simulink model "DSTATCOM (1)"  (R2023b)
settings: Solver=ode5  StartTime=0.0  StopTime=1  FixedStep=50e-8  RelTol=1e-3
InitFcn:
  | v= 400
  | p= 2500
  | q=1500
  | s=2915.47
libraries: spsThreePhaseVIMeasurementLib x11, spsThreePhaseSeriesRLCBranchLib x9, spsThreePhaseSeriesRLCLoadLib x8, spsIGBTDiodeLib x6, slpidlib x4, spsRMSLib x2, spsAlphaBetaZerotodq0Lib x2, spsabctodq0Lib x2, spsSeriesRLCBranchLib x1, simulink x1, spsVoltageMeasurementLib x1, spsabctoAlphaBetaZeroLib x1
settings Model: Creator=prabh  LastModifiedBy=Sandesh

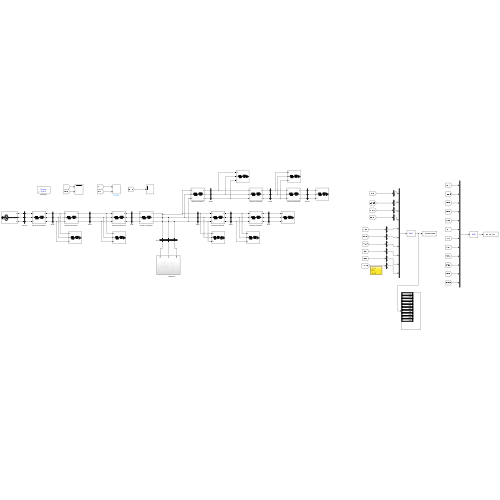
[thumbnail: Simulink's stored preview of the top-level diagram]
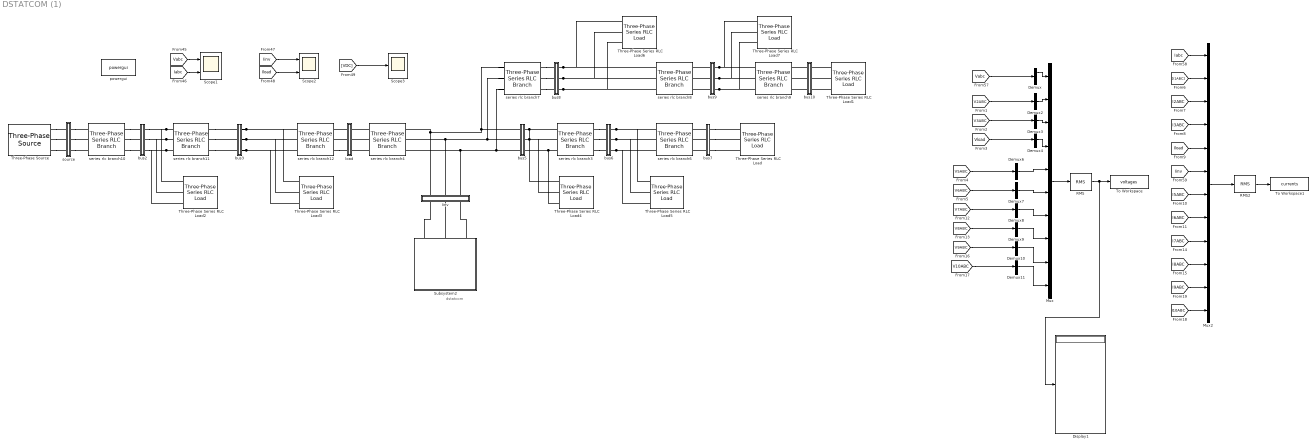
== system DSTATCOM (1) ==
  note: dstatcom
  Demux{,2..4,6..11} (10 alike) : Demux  Outputs=3
  Display1 : Display
  Iinv : Subsystem
  Mux : Mux  Inputs=10
  Mux2 : Mux  Inputs=12
  RMS : spsRMSLib/RMS  TrueRMS=on  Freq=50  RMSInit=0  Ts=0
  RMS2 : spsRMSLib/RMS  TrueRMS=on  Freq=50  RMSInit=0  Ts=0
  Scope1 : Scope  NumInputPorts=2
  Scope2 : Scope  NumInputPorts=2
  Scope3 : Scope
  Subsystem2 : Subsystem
  Three-Phase Series RLC Load{,1..3,5..7} (7 alike) : spsThreePhaseSeriesRLCLoadLib/Three-Phase Series RLC Load  LConnTagsString=A|B|C  Configuration=Y (grounded)  NominalVoltage=v  Vabc=[1e3 1e3 1e3]  Vabcp=[1e3 1e3 1e3]  NominalFrequency=50  UnbalancedPower=off  ActivePower=p  InductivePower=q  CapacitivePower=0  Pabc=[10e3 9e3 11e3]  QLabc=[100 90 110]  QCabc=[100 90 110]  Pabcp=[10e3 9e3 11e3]  QLabcp=[100 90 110]  QCabcp=[100 90 110]  Measurements=None  LoadType=constant PQ
  Three-Phase Series RLC Load4 : spsThreePhaseSeriesRLCLoadLib/Three-Phase Series RLC Load  LConnTagsString=A|B|C  Configuration=Y (grounded)  NominalVoltage=v  Vabc=[1e3 1e3 1e3]  Vabcp=[1e3 1e3 1e3]  NominalFrequency=50  UnbalancedPower=off  ActivePower=p  InductivePower=q  CapacitivePower=q  Pabc=[10e3 9e3 11e3]  QLabc=[100 90 110]  QCabc=[100 90 110]  Pabcp=[10e3 9e3 11e3]  QLabcp=[100 90 110]  QCabcp=[100 90 110]  Measurements=None  LoadType=constant PQ
  Three-Phase Source : spsThreePhaseSourceLib/Three-Phase Source  InternalConnection=Yg  VoltagePhases=off  Voltage=400  PhaseAngle=0  Voltage_phases=[25e3 25e3 25e3]/sqrt(3)  PhaseAngles_phases=[0 -120 +120]  Frequency=50  NonIdealSource=off  SpecifyImpedance=off  Resistance=0.8929  Inductance=16.58e-3  ShortCircuitLevel=100e6  BaseVoltage=25e3  XRratio=7  BusType=swing  Pref=10e3  Qref=0  Prefabc=[10e3, 10e3, 10e3]  Qrefabc=[0, 0, 0]  Qmin=-inf  Qmax=inf
  To Workspace : ToWorkspace  VariableName=voltages  SampleTime=-1
      settings: MaxDataPoints=1
  To Workspace1 : ToWorkspace  VariableName=currents  SampleTime=-1
      settings: MaxDataPoints=1
  bus10 : Subsystem
  bus2 : Subsystem
  bus3 : Subsystem
  bus5 : Subsystem
  bus6 : Subsystem
  bus7 : Subsystem
  bus8 : Subsystem
  bus9 : Subsystem
  load : Subsystem
  powergui : sps_lib/powergui  Priority=1  SimulationMode=Discrete  SampleTime=50e-6  frequency=60  Iterations=50  frequencyindice=0  Pbase=100e6  ErrMax=1e-4  UnitsV=kV  UnitsW=MW  buscounter=0  FunctionMessages=off  echomessages=off  EnableUseOfTLC=off  CurrentSourceSwitches=off  DisableSnubberDevices=off  DisableRonSwitches=off  DisableVfSwitches=off  DisplayEquations=off  AutomaticDiscreteSolvers=off  SolverType=Tustin/Backward Euler (TBE)  Interpol=off  ExternalGateDelay=off  methode=off  Ts=100  x0status=blocks  SPID=on  SwTol=0  HookPort=off  NonlinearTolerance=1e-4  nMaxIteration=100  ContinueOnMaxIteration=off  RestoreLinks=warning  ResistiveCurrentMeasurement=off  Frange=[0:2:500]  Ylog=off  Xlog=on  ShowGrid=off  save=off  variable=ZData  structure=0  ZoomFFT=off  StartTime=0.0  cycles=1  DisplayStyle=1  fundamental=60  FreqAxis=off  MaxFrequency=1000  frequencyindicesteady=1  RmsSteady=1  display=off
  series rlc branch10 : spsThreePhaseSeriesRLCBranchLib/Three-Phase Series RLC Branch  LConnTagsString=A|B|C  RConnTagsString=A|B|C  BranchType=RL  Resistance=0.3  Inductance=0.00027  Capacitance=0  Measurements=None
  series rlc branch11 : spsThreePhaseSeriesRLCBranchLib/Three-Phase Series RLC Branch  LConnTagsString=A|B|C  RConnTagsString=A|B|C  BranchType=RL  Resistance=.3  Inductance=.00177  Capacitance=0  Measurements=None
  series rlc branch12 : spsThreePhaseSeriesRLCBranchLib/Three-Phase Series RLC Branch  LConnTagsString=A|B|C  RConnTagsString=A|B|C  BranchType=RL  Resistance=.3  Inductance=.00218  Capacitance=0  Measurements=None
  series rlc branch3 : spsThreePhaseSeriesRLCBranchLib/Three-Phase Series RLC Branch  LConnTagsString=A|B|C  RConnTagsString=A|B|C  BranchType=RL  Resistance=.36  Inductance=.000821  Capacitance=0  Measurements=None
  series rlc branch4 : spsThreePhaseSeriesRLCBranchLib/Three-Phase Series RLC Branch  LConnTagsString=A|B|C  RConnTagsString=A|B|C  BranchType=RL  Resistance=.77  Inductance=.00218  Capacitance=0  Measurements=None
  series rlc branch6 : spsThreePhaseSeriesRLCBranchLib/Three-Phase Series RLC Branch  LConnTagsString=A|B|C  RConnTagsString=A|B|C  BranchType=RL  Resistance=.3  Inductance=.00068  Capacitance=0  Measurements=None
  series rlc branch7 : spsThreePhaseSeriesRLCBranchLib/Three-Phase Series RLC Branch  LConnTagsString=A|B|C  RConnTagsString=A|B|C  BranchType=RL  Resistance=.18  Inductance=.00041  Capacitance=0  Measurements=None
  series rlc branch8 : spsThreePhaseSeriesRLCBranchLib/Three-Phase Series RLC Branch  LConnTagsString=A|B|C  RConnTagsString=A|B|C  BranchType=RL  Resistance=.12  Inductance=.00027  Capacitance=0  Measurements=None
  series rlc branch9 : spsThreePhaseSeriesRLCBranchLib/Three-Phase Series RLC Branch  LConnTagsString=A|B|C  RConnTagsString=A|B|C  BranchType=RL  Resistance=.6  Inductance=.00136  Capacitance=0  Measurements=None
  source : Subsystem
  wires:
  Mux2/1 -> RMS2/1
  RMS/1 -> Display1/1, To Workspace/1
  RMS2/1 -> To Workspace1/1
  [Iabc] -> Scope1/2
  [Vabc] -> Scope1/1
  [Iinv] -> Scope2/1
  [Iload] -> Scope2/2
  [VDC] -> Scope3/1
  [Vabc] -> Demux/1
  [V2ABC] -> Demux2/1
  [V3ABC] -> Demux3/1
  [Vload] -> Demux4/1
  [V5ABC] -> Demux6/1
  [V6ABC] -> Demux7/1
  [V7ABC] -> Demux8/1
  [V8ABC] -> Demux9/1
  [V9ABC] -> Demux10/1
  [V10ABC] -> Demux11/1
  [Iabc] -> Mux2/1
  [I1ABC] -> Mux2/2
  [I2ABC] -> Mux2/3
  [I3ABC] -> Mux2/4
  [Iload] -> Mux2/5
  [Iinv] -> Mux2/6
  [I5ABC] -> Mux2/7
  [I6ABC] -> Mux2/8
  [I7ABC] -> Mux2/9
  [I8ABC] -> Mux2/10
  [I9ABC] -> Mux2/11
  [I10ABC] -> Mux2/12
  Mux/1 -> RMS/1
  Demux/1 -> Mux/1
  Demux2/2 -> Mux/2
  Demux3/2 -> Mux/3
  Demux4/2 -> Mux/4
  Demux6/2 -> Mux/5
  Demux7/2 -> Mux/6
  Demux8/2 -> Mux/7
  Demux9/2 -> Mux/8
  Demux10/2 -> Mux/9
  Demux11/2 -> Mux/10
  connections:
  source/RConn1 -- series rlc branch10/LConn1
  source/RConn2 -- series rlc branch10/LConn2
  source/RConn3 -- series rlc branch10/LConn3
  Three-Phase Source/RConn2 -- source/LConn2
  Three-Phase Source/RConn1 -- source/LConn1
  Three-Phase Source/RConn3 -- source/LConn3
  series rlc branch4/LConn2 -- load/RConn2
  series rlc branch4/LConn1 -- load/RConn1
  series rlc branch4/LConn3 -- load/RConn3
  bus8/RConn1 -- series rlc branch8/LConn1 -- Three-Phase Series RLC Load6/LConn1
  bus9/RConn3 -- series rlc branch9/LConn3 -- Three-Phase Series RLC Load7/LConn3
  bus9/RConn2 -- series rlc branch9/LConn2 -- Three-Phase Series RLC Load7/LConn2
  bus9/RConn1 -- series rlc branch9/LConn1 -- Three-Phase Series RLC Load7/LConn1
  bus8/RConn3 -- series rlc branch8/LConn3 -- Three-Phase Series RLC Load6/LConn3
  bus8/RConn2 -- series rlc branch8/LConn2 -- Three-Phase Series RLC Load6/LConn2
  bus9/LConn2 -- series rlc branch8/RConn2
  bus9/LConn1 -- series rlc branch8/RConn1
  Three-Phase Series RLC Load1/LConn3 -- bus10/RConn3
  Three-Phase Series RLC Load1/LConn1 -- bus10/RConn1
  bus10/LConn1 -- series rlc branch9/RConn1
  series rlc branch7/RConn3 -- bus8/LConn3
  bus9/LConn3 -- series rlc branch8/RConn3
  bus10/LConn2 -- series rlc branch9/RConn2
  Three-Phase Series RLC Load1/LConn2 -- bus10/RConn2
  series rlc branch7/RConn1 -- bus8/LConn1
  series rlc branch7/RConn2 -- bus8/LConn2
  bus10/LConn3 -- series rlc branch9/RConn3
  bus6/RConn1 -- series rlc branch6/LConn1 -- Three-Phase Series RLC Load5/LConn1
  bus6/RConn3 -- series rlc branch6/LConn3 -- Three-Phase Series RLC Load5/LConn3
  bus5/RConn1 -- series rlc branch3/LConn1 -- Three-Phase Series RLC Load4/LConn1
  bus6/RConn2 -- series rlc branch6/LConn2 -- Three-Phase Series RLC Load5/LConn2
  Three-Phase Series RLC Load4/LConn3 -- series rlc branch3/LConn3 -- bus5/RConn3
  bus5/RConn2 -- series rlc branch3/LConn2 -- Three-Phase Series RLC Load4/LConn2
  bus7/RConn3 -- Three-Phase Series RLC Load/LConn3
  series rlc branch3/RConn3 -- bus6/LConn3
  bus7/RConn1 -- Three-Phase Series RLC Load/LConn1
  bus7/RConn2 -- Three-Phase Series RLC Load/LConn2
  bus7/LConn1 -- series rlc branch6/RConn1
  series rlc branch3/RConn1 -- bus6/LConn1
  series rlc branch7/LConn1 -- series rlc branch4/RConn1 -- Iinv/LConn1 -- bus5/LConn1
  series rlc branch7/LConn3 -- bus5/LConn3 -- Iinv/LConn3 -- series rlc branch4/RConn3
  bus7/LConn2 -- series rlc branch6/RConn2
  bus7/LConn3 -- series rlc branch6/RConn3
  series rlc branch3/RConn2 -- bus6/LConn2
  series rlc branch7/LConn2 -- bus5/LConn2 -- Iinv/LConn2 -- series rlc branch4/RConn2
  series rlc branch11/LConn3 -- bus2/RConn3 -- Three-Phase Series RLC Load2/LConn3
  series rlc branch11/LConn1 -- bus2/RConn1 -- Three-Phase Series RLC Load2/LConn1
  series rlc branch11/LConn2 -- bus2/RConn2 -- Three-Phase Series RLC Load2/LConn2
  bus3/RConn3 -- series rlc branch12/LConn3 -- Three-Phase Series RLC Load3/LConn3
  bus3/RConn2 -- series rlc branch12/LConn2 -- Three-Phase Series RLC Load3/LConn2
  bus3/RConn1 -- series rlc branch12/LConn1 -- Three-Phase Series RLC Load3/LConn1
  series rlc branch11/RConn3 -- bus3/LConn3
  series rlc branch11/RConn1 -- bus3/LConn1
  series rlc branch10/RConn1 -- bus2/LConn1
  series rlc branch10/RConn2 -- bus2/LConn2
  series rlc branch10/RConn3 -- bus2/LConn3
  series rlc branch11/RConn2 -- bus3/LConn2
  load/LConn1 -- series rlc branch12/RConn1
  load/LConn2 -- series rlc branch12/RConn2
  series rlc branch12/RConn3 -- load/LConn3
  Subsystem2/LConn1 -- Iinv/RConn1
  Subsystem2/LConn2 -- Iinv/RConn2
  Subsystem2/LConn3 -- Iinv/RConn3

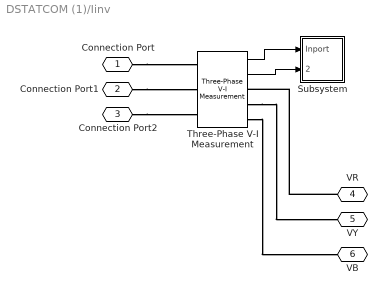
== system DSTATCOM (1)/Iinv ==
  Subsystem : Subsystem
  Three-Phase V-I Measurement : spsThreePhaseVIMeasurementLib/Three-Phase V-I Measurement  VoltageMeasurement=phase-to-ground  SetLabelV=off  LabelV=Vabc  Vpu=off  VpuLL=off  CurrentMeasurement=yes  SetLabelI=off  LabelI=Iabc  Ipu=off  Pbase=100e6  Vbase=500e3  OutputType=Complex  PhasorSimulation=off  PSBequivalent=0
  Connection Port : PMIOPort  Side=Left
  Connection Port1 : PMIOPort  Port=2  Side=Left
  Connection Port2 : PMIOPort  Port=3  Side=Left
  VR : PMIOPort  Port=4  Side=Right
  VY : PMIOPort  Port=5  Side=Right
  VB : PMIOPort  Port=6  Side=Right
  wires:
  Three-Phase V-I Measurement/1 -> Subsystem/1(Inport)
  Three-Phase V-I Measurement/2 -> Subsystem/2(Inport1)
  connections:
  Connection Port/RConn1 -- Three-Phase V-I Measurement/LConn1
  Connection Port1/RConn1 -- Three-Phase V-I Measurement/LConn2
  Connection Port2/RConn1 -- Three-Phase V-I Measurement/LConn3
  VR/RConn1 -- Three-Phase V-I Measurement/RConn1
  Three-Phase V-I Measurement/RConn2 -- VY/RConn1
  Three-Phase V-I Measurement/RConn3 -- VB/RConn1

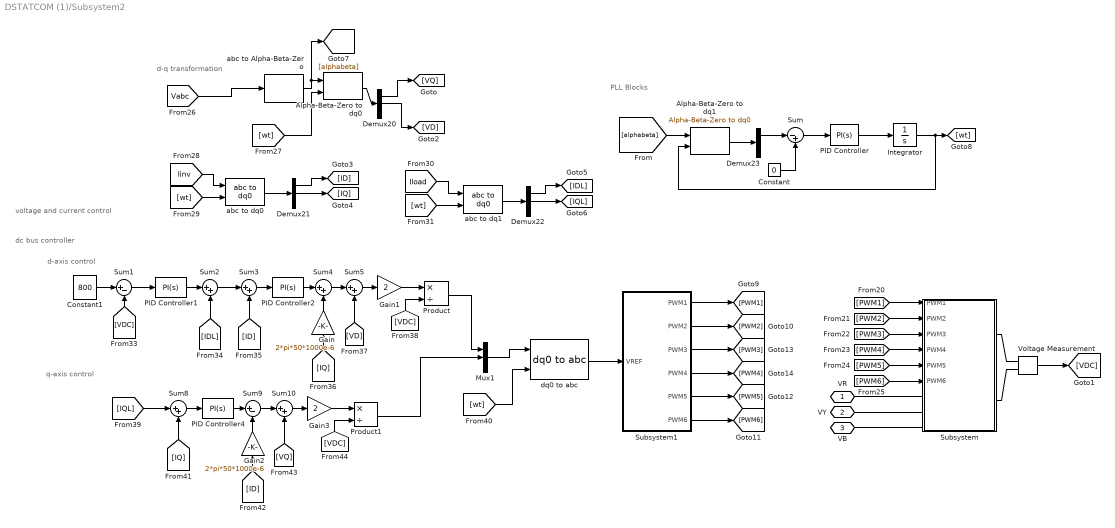
== system DSTATCOM (1)/Subsystem2 ==
  note: q-axis control
  note: d-axis control
  note: dc bus controller
  note: voltage and current control
  note: PLL Blocks
  note: d-q transformation
  Alpha-Beta-Zero to dq0 : spsAlphaBetaZerotodq0Lib/Alpha-Beta-Zero to dq0  Alignment=90 degrees behind phase A axis
  Alpha-Beta-Zero to dq1 : spsAlphaBetaZerotodq0Lib/Alpha-Beta-Zero to dq0  Alignment=90 degrees behind phase A axis
  Constant : Constant  Value=0
  Constant1 : Constant  Value=800
  Demux{20..23} (4 alike) : Demux  Outputs=3
  Gain : Gain  Gain=2*pi*50*1000e-6
  Gain1 : Gain  Gain=2
  Gain2 : Gain  Gain=2*pi*50*1000e-6
  Gain3 : Gain  Gain=2
  Integrator : Integrator
  Mux1 : Mux  Inputs=3
  PID Controller : slpidlib/PID Controller  Controller=PI  Form=Parallel  TimeDomain=Continuous-time  UseExternalTs=off  SampleTime=-1  IntegratorMethod=Forward Euler  FilterMethod=Forward Euler  ControllerParametersSource=internal  P=10  I=50000  UseKiTs=off  D=0  N=100  UseFilter=on  TunerSelectOption=Transfer Function Based (PID Tuner App)  InitialConditionSource=internal  InitialConditionForIntegrator=0  InitialConditionForFilter=0  DifferentiatorICPrevScaledInput=0  ExternalReset=none  TrackingMode=off  Kt=1  LimitOutput=off  SatLimitsSource=internal  UpperSaturationLimit=inf  LowerSaturationLimit=-inf  LinearizeAsGain=on  AntiWindupMode=none  Kb=1  LimitIntegrator=off  UpperIntegratorSaturationLimit=inf  LowerIntegratorSaturationLimit=-inf  POutMin=[]  POutMax=[]  IOutMin=[]  IOutMax=[]  DOutMin=[]  DOutMax=[]  NOutMin=[]  NOutMax=[]  SumOutMin=[]  SumOutMax=[]  SaturationOutMin=[]  SaturationOutMax=[]  PParamMin=[]  PParamMax=[]  IParamMin=[]  IParamMax=[]  DParamMin=[]  DParamMax=[]  NParamMin=[]  NParamMax=[]  KbParamMin=[]  KbParamMax=[]  KtParamMin=[]  KtParamMax=[]  KbOutMin=[]  KbOutMax=[]  KtOutMin=[]  KtOutMax=[]  IntegratorOutMin=[]  IntegratorOutMax=[]  FilterOutMin=[]  FilterOutMax=[]  SumI1OutMin=[]  SumI1OutMax=[]  SumI2OutMin=[]  SumI2OutMax=[]  SumI3OutMin=[]  SumI3OutMax=[]  SumI4OutMin=[]  SumI4OutMax=[]  SumDOutMin=[]  SumDOutMax=[]  DifferentiatorOutMin=[]  DifferentiatorOutMax=[]  FilterDiffOutCoefMin=[]  FilterDiffOutCoefMax=[]  ReciprocalOutMin=[]  ReciprocalOutMax=[]  SumDenOutMin=[]  SumDenOutMax=[]  SumNumOutMin=[]  SumNumOutMax=[]  DivideOutMin=[]  DivideOutMax=[]  UdiffTsProdOutMin=[]  UdiffTsProdOutMax=[]  NTsProdOutMin=[]  NTsProdOutMax=[]  UintegralTsProdOutMin=[]  UintegralTsProdOutMax=[]  UngainTsProdOutMin=[]  UngainTsProdOutMax=[]  ClampingZeroOutDataTypeStr=Inherit: Inherit via back propagation  ClampingZeroOutMin=[]  ClampingZeroOutMax=[]  FilterDenConstantOutDataTypeStr=Inherit: Inherit via back propagation  FilterDenConstantOutMin=[]  FilterDenConstantOutMax=[]  PCopyOutDataTypeStr=Inherit: Inherit via back propagation  PCopyOutMin=[]  PCopyOutMax=[]  NCopyOutDataTypeStr=Inherit: Inherit via back propagation  NCopyOutMin=[]  NCopyOutMax=[]  IntegratorContinuousStateAttributes=''  IntegratorStateMustResolveToSignalObject=off  IntegratorRTWStateStorageClass=Auto  FilterContinuousStateAttributes=''  FilterStateMustResolveToSignalObject=off  FilterRTWStateStorageClass=Auto  ParallelPVariant=InternalParameters  IdealPVariant=Disabled  IVariant=InternalParameters  DVariant=Disabled  IntegratorVariant=Continuous  SatVariant=Disabled  AWVariant=Passthrough  PCopyVariant=Disabled  TRVariant=Disabled  FdbkBlocksVariant=Forward  IdealPFdbkVariant=Disabled  SatFdbkVariant=Disabled  DerivativeFilterVariant=Disabled  NVariant=Disabled  NCopyVariant=Disabled_SignalSpec  FilterICVariant=Disabled  IntegratorICVariant=InternalICs  ExternalResetVariant=Disabled  TRSumVariant=Passthrough  SumFdbkVariant=Disabled  SumVariant=Sum_PI  TsampFilterVariant=InternalTs  TsampNgainVariant=Passthrough  TsampIntegralVariant=Disabled_SignalSpec  ExternalSaturationOutDataTypeStr=Inherit: Same as second input
  PID Controller1 : slpidlib/PID Controller  Controller=PI  Form=Parallel  TimeDomain=Continuous-time  UseExternalTs=off  SampleTime=-1  IntegratorMethod=Forward Euler  FilterMethod=Forward Euler  ControllerParametersSource=internal  P=5  I=200  UseKiTs=off  D=0  N=100  UseFilter=on  TunerSelectOption=Transfer Function Based (PID Tuner App)  InitialConditionSource=internal  InitialConditionForIntegrator=0  InitialConditionForFilter=0  DifferentiatorICPrevScaledInput=0  ExternalReset=none  TrackingMode=off  Kt=1  LimitOutput=off  SatLimitsSource=internal  UpperSaturationLimit=inf  LowerSaturationLimit=-inf  LinearizeAsGain=on  AntiWindupMode=none  Kb=1  LimitIntegrator=off  UpperIntegratorSaturationLimit=inf  LowerIntegratorSaturationLimit=-inf  POutMin=[]  POutMax=[]  IOutMin=[]  IOutMax=[]  DOutMin=[]  DOutMax=[]  NOutMin=[]  NOutMax=[]  SumOutMin=[]  SumOutMax=[]  SaturationOutMin=[]  SaturationOutMax=[]  PParamMin=[]  PParamMax=[]  IParamMin=[]  IParamMax=[]  DParamMin=[]  DParamMax=[]  NParamMin=[]  NParamMax=[]  KbParamMin=[]  KbParamMax=[]  KtParamMin=[]  KtParamMax=[]  KbOutMin=[]  KbOutMax=[]  KtOutMin=[]  KtOutMax=[]  IntegratorOutMin=[]  IntegratorOutMax=[]  FilterOutMin=[]  FilterOutMax=[]  SumI1OutMin=[]  SumI1OutMax=[]  SumI2OutMin=[]  SumI2OutMax=[]  SumI3OutMin=[]  SumI3OutMax=[]  SumI4OutMin=[]  SumI4OutMax=[]  SumDOutMin=[]  SumDOutMax=[]  DifferentiatorOutMin=[]  DifferentiatorOutMax=[]  FilterDiffOutCoefMin=[]  FilterDiffOutCoefMax=[]  ReciprocalOutMin=[]  ReciprocalOutMax=[]  SumDenOutMin=[]  SumDenOutMax=[]  SumNumOutMin=[]  SumNumOutMax=[]  DivideOutMin=[]  DivideOutMax=[]  UdiffTsProdOutMin=[]  UdiffTsProdOutMax=[]  NTsProdOutMin=[]  NTsProdOutMax=[]  UintegralTsProdOutMin=[]  UintegralTsProdOutMax=[]  UngainTsProdOutMin=[]  UngainTsProdOutMax=[]  ClampingZeroOutDataTypeStr=Inherit: Inherit via back propagation  ClampingZeroOutMin=[]  ClampingZeroOutMax=[]  FilterDenConstantOutDataTypeStr=Inherit: Inherit via back propagation  FilterDenConstantOutMin=[]  FilterDenConstantOutMax=[]  PCopyOutDataTypeStr=Inherit: Inherit via back propagation  PCopyOutMin=[]  PCopyOutMax=[]  NCopyOutDataTypeStr=Inherit: Inherit via back propagation  NCopyOutMin=[]  NCopyOutMax=[]  IntegratorContinuousStateAttributes=''  IntegratorStateMustResolveToSignalObject=off  IntegratorRTWStateStorageClass=Auto  FilterContinuousStateAttributes=''  FilterStateMustResolveToSignalObject=off  FilterRTWStateStorageClass=Auto  ParallelPVariant=InternalParameters  IdealPVariant=Disabled  IVariant=InternalParameters  DVariant=Disabled  IntegratorVariant=Continuous  SatVariant=Disabled  AWVariant=Passthrough  PCopyVariant=Disabled  TRVariant=Disabled  FdbkBlocksVariant=Forward  IdealPFdbkVariant=Disabled  SatFdbkVariant=Disabled  DerivativeFilterVariant=Disabled  NVariant=Disabled  NCopyVariant=Disabled_SignalSpec  FilterICVariant=Disabled  IntegratorICVariant=InternalICs  ExternalResetVariant=Disabled  TRSumVariant=Passthrough  SumFdbkVariant=Disabled  SumVariant=Sum_PI  TsampFilterVariant=InternalTs  TsampNgainVariant=Passthrough  TsampIntegralVariant=Disabled_SignalSpec  ExternalSaturationOutDataTypeStr=Inherit: Same as second input
  PID Controller2 : slpidlib/PID Controller  Controller=PI  Form=Parallel  TimeDomain=Continuous-time  UseExternalTs=off  SampleTime=-1  IntegratorMethod=Forward Euler  FilterMethod=Forward Euler  ControllerParametersSource=internal  P=25  I=500  UseKiTs=off  D=0  N=100  UseFilter=on  TunerSelectOption=Transfer Function Based (PID Tuner App)  InitialConditionSource=internal  InitialConditionForIntegrator=0  InitialConditionForFilter=0  DifferentiatorICPrevScaledInput=0  ExternalReset=none  TrackingMode=off  Kt=1  LimitOutput=off  SatLimitsSource=internal  UpperSaturationLimit=inf  LowerSaturationLimit=-inf  LinearizeAsGain=on  AntiWindupMode=none  Kb=1  LimitIntegrator=off  UpperIntegratorSaturationLimit=inf  LowerIntegratorSaturationLimit=-inf  POutMin=[]  POutMax=[]  IOutMin=[]  IOutMax=[]  DOutMin=[]  DOutMax=[]  NOutMin=[]  NOutMax=[]  SumOutMin=[]  SumOutMax=[]  SaturationOutMin=[]  SaturationOutMax=[]  PParamMin=[]  PParamMax=[]  IParamMin=[]  IParamMax=[]  DParamMin=[]  DParamMax=[]  NParamMin=[]  NParamMax=[]  KbParamMin=[]  KbParamMax=[]  KtParamMin=[]  KtParamMax=[]  KbOutMin=[]  KbOutMax=[]  KtOutMin=[]  KtOutMax=[]  IntegratorOutMin=[]  IntegratorOutMax=[]  FilterOutMin=[]  FilterOutMax=[]  SumI1OutMin=[]  SumI1OutMax=[]  SumI2OutMin=[]  SumI2OutMax=[]  SumI3OutMin=[]  SumI3OutMax=[]  SumI4OutMin=[]  SumI4OutMax=[]  SumDOutMin=[]  SumDOutMax=[]  DifferentiatorOutMin=[]  DifferentiatorOutMax=[]  FilterDiffOutCoefMin=[]  FilterDiffOutCoefMax=[]  ReciprocalOutMin=[]  ReciprocalOutMax=[]  SumDenOutMin=[]  SumDenOutMax=[]  SumNumOutMin=[]  SumNumOutMax=[]  DivideOutMin=[]  DivideOutMax=[]  UdiffTsProdOutMin=[]  UdiffTsProdOutMax=[]  NTsProdOutMin=[]  NTsProdOutMax=[]  UintegralTsProdOutMin=[]  UintegralTsProdOutMax=[]  UngainTsProdOutMin=[]  UngainTsProdOutMax=[]  ClampingZeroOutDataTypeStr=Inherit: Inherit via back propagation  ClampingZeroOutMin=[]  ClampingZeroOutMax=[]  FilterDenConstantOutDataTypeStr=Inherit: Inherit via back propagation  FilterDenConstantOutMin=[]  FilterDenConstantOutMax=[]  PCopyOutDataTypeStr=Inherit: Inherit via back propagation  PCopyOutMin=[]  PCopyOutMax=[]  NCopyOutDataTypeStr=Inherit: Inherit via back propagation  NCopyOutMin=[]  NCopyOutMax=[]  IntegratorContinuousStateAttributes=''  IntegratorStateMustResolveToSignalObject=off  IntegratorRTWStateStorageClass=Auto  FilterContinuousStateAttributes=''  FilterStateMustResolveToSignalObject=off  FilterRTWStateStorageClass=Auto  ParallelPVariant=InternalParameters  IdealPVariant=Disabled  IVariant=InternalParameters  DVariant=Disabled  IntegratorVariant=Continuous  SatVariant=Disabled  AWVariant=Passthrough  PCopyVariant=Disabled  TRVariant=Disabled  FdbkBlocksVariant=Forward  IdealPFdbkVariant=Disabled  SatFdbkVariant=Disabled  DerivativeFilterVariant=Disabled  NVariant=Disabled  NCopyVariant=Disabled_SignalSpec  FilterICVariant=Disabled  IntegratorICVariant=InternalICs  ExternalResetVariant=Disabled  TRSumVariant=Passthrough  SumFdbkVariant=Disabled  SumVariant=Sum_PI  TsampFilterVariant=InternalTs  TsampNgainVariant=Passthrough  TsampIntegralVariant=Disabled_SignalSpec  ExternalSaturationOutDataTypeStr=Inherit: Same as second input
  PID Controller4 : slpidlib/PID Controller  Controller=PI  Form=Parallel  TimeDomain=Continuous-time  UseExternalTs=off  SampleTime=-1  IntegratorMethod=Forward Euler  FilterMethod=Forward Euler  ControllerParametersSource=internal  P=25  I=500  UseKiTs=off  D=0  N=100  UseFilter=on  TunerSelectOption=Transfer Function Based (PID Tuner App)  InitialConditionSource=internal  InitialConditionForIntegrator=0  InitialConditionForFilter=0  DifferentiatorICPrevScaledInput=0  ExternalReset=none  TrackingMode=off  Kt=1  LimitOutput=off  SatLimitsSource=internal  UpperSaturationLimit=inf  LowerSaturationLimit=-inf  LinearizeAsGain=on  AntiWindupMode=none  Kb=1  LimitIntegrator=off  UpperIntegratorSaturationLimit=inf  LowerIntegratorSaturationLimit=-inf  POutMin=[]  POutMax=[]  IOutMin=[]  IOutMax=[]  DOutMin=[]  DOutMax=[]  NOutMin=[]  NOutMax=[]  SumOutMin=[]  SumOutMax=[]  SaturationOutMin=[]  SaturationOutMax=[]  PParamMin=[]  PParamMax=[]  IParamMin=[]  IParamMax=[]  DParamMin=[]  DParamMax=[]  NParamMin=[]  NParamMax=[]  KbParamMin=[]  KbParamMax=[]  KtParamMin=[]  KtParamMax=[]  KbOutMin=[]  KbOutMax=[]  KtOutMin=[]  KtOutMax=[]  IntegratorOutMin=[]  IntegratorOutMax=[]  FilterOutMin=[]  FilterOutMax=[]  SumI1OutMin=[]  SumI1OutMax=[]  SumI2OutMin=[]  SumI2OutMax=[]  SumI3OutMin=[]  SumI3OutMax=[]  SumI4OutMin=[]  SumI4OutMax=[]  SumDOutMin=[]  SumDOutMax=[]  DifferentiatorOutMin=[]  DifferentiatorOutMax=[]  FilterDiffOutCoefMin=[]  FilterDiffOutCoefMax=[]  ReciprocalOutMin=[]  ReciprocalOutMax=[]  SumDenOutMin=[]  SumDenOutMax=[]  SumNumOutMin=[]  SumNumOutMax=[]  DivideOutMin=[]  DivideOutMax=[]  UdiffTsProdOutMin=[]  UdiffTsProdOutMax=[]  NTsProdOutMin=[]  NTsProdOutMax=[]  UintegralTsProdOutMin=[]  UintegralTsProdOutMax=[]  UngainTsProdOutMin=[]  UngainTsProdOutMax=[]  ClampingZeroOutDataTypeStr=Inherit: Inherit via back propagation  ClampingZeroOutMin=[]  ClampingZeroOutMax=[]  FilterDenConstantOutDataTypeStr=Inherit: Inherit via back propagation  FilterDenConstantOutMin=[]  FilterDenConstantOutMax=[]  PCopyOutDataTypeStr=Inherit: Inherit via back propagation  PCopyOutMin=[]  PCopyOutMax=[]  NCopyOutDataTypeStr=Inherit: Inherit via back propagation  NCopyOutMin=[]  NCopyOutMax=[]  IntegratorContinuousStateAttributes=''  IntegratorStateMustResolveToSignalObject=off  IntegratorRTWStateStorageClass=Auto  FilterContinuousStateAttributes=''  FilterStateMustResolveToSignalObject=off  FilterRTWStateStorageClass=Auto  ParallelPVariant=InternalParameters  IdealPVariant=Disabled  IVariant=InternalParameters  DVariant=Disabled  IntegratorVariant=Continuous  SatVariant=Disabled  AWVariant=Passthrough  PCopyVariant=Disabled  TRVariant=Disabled  FdbkBlocksVariant=Forward  IdealPFdbkVariant=Disabled  SatFdbkVariant=Disabled  DerivativeFilterVariant=Disabled  NVariant=Disabled  NCopyVariant=Disabled_SignalSpec  FilterICVariant=Disabled  IntegratorICVariant=InternalICs  ExternalResetVariant=Disabled  TRSumVariant=Passthrough  SumFdbkVariant=Disabled  SumVariant=Sum_PI  TsampFilterVariant=InternalTs  TsampNgainVariant=Passthrough  TsampIntegralVariant=Disabled_SignalSpec  ExternalSaturationOutDataTypeStr=Inherit: Same as second input
  Product : Product  Inputs=*/
  Product1 : Product  Inputs=*/
  Subsystem : Subsystem
  Subsystem1 : Subsystem
  Sum : Sum  Inputs=|-+
  Sum1 : Sum  Inputs=|+-
  Sum{2..5,8,10} (6 alike) : Sum  Inputs=|++
  Sum9 : Sum  Inputs=|+-
  Voltage Measurement : spsVoltageMeasurementLib/Voltage Measurement  PhasorSimulation=off  OutputType=Complex  PSBequivalent=0
  abc to Alpha-Beta-Zero : spsabctoAlphaBetaZeroLib/abc to Alpha-Beta-Zero
  abc to dq0 : spsabctodq0Lib/abc to dq0  Alignment=90 degrees behind phase A axis
  abc to dq1 : spsabctodq0Lib/abc to dq0  Alignment=90 degrees behind phase A axis
  dq0 to abc : spsdq0toabcLib/dq0 to abc  Alignment=90 degrees behind phase A axis
  VR : PMIOPort  Side=Left
  VY : PMIOPort  Port=2  Side=Left
  VB : PMIOPort  Port=3  Side=Left
  wires:
  [IQ] -> Sum8/2
  Gain3/1 -> Product1/1
  [PWM6] -> Subsystem/6(PWM6)
  Subsystem1/1(PWM1) -> [PWM1]
  Demux21/1 -> [ID]
  PID Controller/1 -> Integrator/1
  abc to dq1/1 -> Demux22/1
  Voltage Measurement/1 -> [VDC]
  [PWM2] -> Subsystem/2(PWM2)
  Demux22/1 -> [IDL]
  Sum1/1 -> PID Controller1/1
  [Vabc] -> abc to Alpha-Beta-Zero/1
  Sum3/1 -> PID Controller2/1
  [VQ] -> Sum10/2
  [VDC] -> Product/2
  [PWM3] -> Subsystem/3(PWM3)
  [VD] -> Sum5/2
  Product/1 -> Mux1/1
  Alpha-Beta-Zero to dq0/1 -> Demux20/1
  [Iload] -> abc to dq1/1
  [wt] -> Alpha-Beta-Zero to dq0/2
  [ID] -> Sum3/2
  [VDC] -> Product1/2
  Sum4/1 -> Sum5/1
  Sum10/1 -> Gain3/1
  [wt] -> abc to dq0/2
  [IDL] -> Sum2/2
  Gain2/1 -> Sum9/2
  [wt] -> abc to dq1/2
  Subsystem1/2(PWM2) -> [PWM2]
  Demux22/2 -> [IQL]
  Subsystem1/5(PWM5) -> [PWM5]
  Alpha-Beta-Zero to dq1/1 -> Demux23/1
  PID Controller1/1 -> Sum2/1
  Demux20/1 -> [VQ]
  [ID] -> Gain2/1
  Sum2/1 -> Sum3/1
  [PWM5] -> Subsystem/5(PWM5)
  [wt] -> dq0 to abc/2
  Demux23/1 -> Sum/1
  PID Controller4/1 -> Sum9/1
  Sum9/1 -> Sum10/1
  Sum/1 -> PID Controller/1
  Sum8/1 -> PID Controller4/1
  Subsystem1/4(PWM4) -> [PWM4]
  Demux20/2 -> [VD]
  Constant1/1 -> Sum1/1
  Sum5/1 -> Gain1/1
  dq0 to abc/1 -> Subsystem1/1(VREF)
  Constant/1 -> Sum/2
  [PWM4] -> Subsystem/4(PWM4)
  [PWM1] -> Subsystem/1(PWM1)
  Gain/1 -> Sum4/2
  [IQL] -> Sum8/1
  Gain1/1 -> Product/1
  [VDC] -> Sum1/2
  Subsystem1/3(PWM3) -> [PWM3]
  Product1/1 -> Mux1/2
  Subsystem1/6(PWM6) -> [PWM6]
  [Iinv] -> abc to dq0/1
  [alphabeta] -> Alpha-Beta-Zero to dq1/1
  PID Controller2/1 -> Sum4/1
  [IQ] -> Gain/1
  Integrator/1 -> Alpha-Beta-Zero to dq1/2, [wt]
  Mux1/1 -> dq0 to abc/1
  Demux21/2 -> [IQ]
  abc to dq0/1 -> Demux21/1
  abc to Alpha-Beta-Zero/1 -> [alphabeta], Alpha-Beta-Zero to dq0/1
  connections:
  Voltage Measurement/LConn1 -- Subsystem/RConn1
  Voltage Measurement/LConn2 -- Subsystem/RConn2
  VB/RConn1 -- Subsystem/LConn3
  VY/RConn1 -- Subsystem/LConn2
  VR/RConn1 -- Subsystem/LConn1

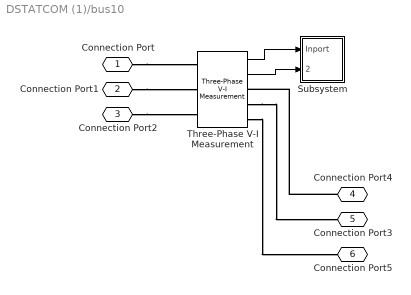
== system DSTATCOM (1)/bus10 ==
  Subsystem : Subsystem
  Three-Phase V-I Measurement : spsThreePhaseVIMeasurementLib/Three-Phase V-I Measurement  VoltageMeasurement=phase-to-ground  SetLabelV=off  LabelV=Vabc  Vpu=off  VpuLL=off  CurrentMeasurement=yes  SetLabelI=off  LabelI=Iabc  Ipu=off  Pbase=100e6  Vbase=500e3  OutputType=Complex  PhasorSimulation=off  PSBequivalent=0
  Connection Port : PMIOPort  Side=Left
  Connection Port1 : PMIOPort  Port=2  Side=Left
  Connection Port2 : PMIOPort  Port=3  Side=Left
  Connection Port4 : PMIOPort  Port=4  Side=Right
  Connection Port3 : PMIOPort  Port=5  Side=Right
  Connection Port5 : PMIOPort  Port=6  Side=Right
  wires:
  Three-Phase V-I Measurement/1 -> Subsystem/1(Inport)
  Three-Phase V-I Measurement/2 -> Subsystem/2(Inport1)
  connections:
  Connection Port/RConn1 -- Three-Phase V-I Measurement/LConn1
  Connection Port1/RConn1 -- Three-Phase V-I Measurement/LConn2
  Connection Port2/RConn1 -- Three-Phase V-I Measurement/LConn3
  Connection Port4/RConn1 -- Three-Phase V-I Measurement/RConn1
  Three-Phase V-I Measurement/RConn2 -- Connection Port3/RConn1
  Three-Phase V-I Measurement/RConn3 -- Connection Port5/RConn1

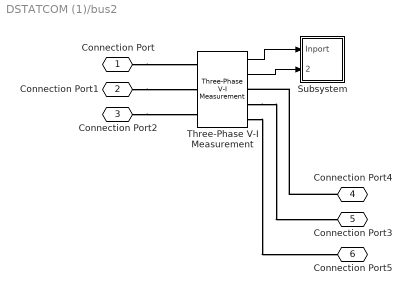
== system DSTATCOM (1)/bus2 ==
  Subsystem : Subsystem
  Three-Phase V-I Measurement : spsThreePhaseVIMeasurementLib/Three-Phase V-I Measurement  VoltageMeasurement=phase-to-ground  SetLabelV=off  LabelV=Vabc  Vpu=off  VpuLL=off  CurrentMeasurement=yes  SetLabelI=off  LabelI=Iabc  Ipu=off  Pbase=100e6  Vbase=500e3  OutputType=Complex  PhasorSimulation=off  PSBequivalent=0
  Connection Port : PMIOPort  Side=Left
  Connection Port1 : PMIOPort  Port=2  Side=Left
  Connection Port2 : PMIOPort  Port=3  Side=Left
  Connection Port4 : PMIOPort  Port=4  Side=Right
  Connection Port3 : PMIOPort  Port=5  Side=Right
  Connection Port5 : PMIOPort  Port=6  Side=Right
  wires:
  Three-Phase V-I Measurement/1 -> Subsystem/1(Inport)
  Three-Phase V-I Measurement/2 -> Subsystem/2(Inport1)
  connections:
  Connection Port/RConn1 -- Three-Phase V-I Measurement/LConn1
  Connection Port1/RConn1 -- Three-Phase V-I Measurement/LConn2
  Connection Port2/RConn1 -- Three-Phase V-I Measurement/LConn3
  Connection Port4/RConn1 -- Three-Phase V-I Measurement/RConn1
  Three-Phase V-I Measurement/RConn2 -- Connection Port3/RConn1
  Three-Phase V-I Measurement/RConn3 -- Connection Port5/RConn1

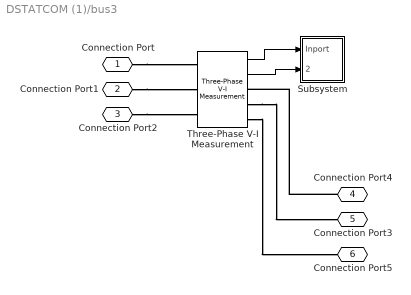
== system DSTATCOM (1)/bus3 ==
  Subsystem : Subsystem
  Three-Phase V-I Measurement : spsThreePhaseVIMeasurementLib/Three-Phase V-I Measurement  VoltageMeasurement=phase-to-ground  SetLabelV=off  LabelV=Vabc  Vpu=off  VpuLL=off  CurrentMeasurement=yes  SetLabelI=off  LabelI=Iabc  Ipu=off  Pbase=100e6  Vbase=500e3  OutputType=Complex  PhasorSimulation=off  PSBequivalent=0
  Connection Port : PMIOPort  Side=Left
  Connection Port1 : PMIOPort  Port=2  Side=Left
  Connection Port2 : PMIOPort  Port=3  Side=Left
  Connection Port4 : PMIOPort  Port=4  Side=Right
  Connection Port3 : PMIOPort  Port=5  Side=Right
  Connection Port5 : PMIOPort  Port=6  Side=Right
  wires:
  Three-Phase V-I Measurement/1 -> Subsystem/1(Inport)
  Three-Phase V-I Measurement/2 -> Subsystem/2(Inport1)
  connections:
  Connection Port/RConn1 -- Three-Phase V-I Measurement/LConn1
  Connection Port1/RConn1 -- Three-Phase V-I Measurement/LConn2
  Connection Port2/RConn1 -- Three-Phase V-I Measurement/LConn3
  Connection Port4/RConn1 -- Three-Phase V-I Measurement/RConn1
  Three-Phase V-I Measurement/RConn2 -- Connection Port3/RConn1
  Three-Phase V-I Measurement/RConn3 -- Connection Port5/RConn1

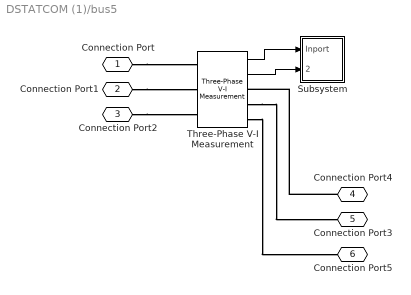
== system DSTATCOM (1)/bus5 ==
  Subsystem : Subsystem
  Three-Phase V-I Measurement : spsThreePhaseVIMeasurementLib/Three-Phase V-I Measurement  VoltageMeasurement=phase-to-ground  SetLabelV=off  LabelV=Vabc  Vpu=off  VpuLL=off  CurrentMeasurement=yes  SetLabelI=off  LabelI=Iabc  Ipu=off  Pbase=100e6  Vbase=500e3  OutputType=Complex  PhasorSimulation=off  PSBequivalent=0
  Connection Port : PMIOPort  Side=Left
  Connection Port1 : PMIOPort  Port=2  Side=Left
  Connection Port2 : PMIOPort  Port=3  Side=Left
  Connection Port4 : PMIOPort  Port=4  Side=Right
  Connection Port3 : PMIOPort  Port=5  Side=Right
  Connection Port5 : PMIOPort  Port=6  Side=Right
  wires:
  Three-Phase V-I Measurement/1 -> Subsystem/1(Inport)
  Three-Phase V-I Measurement/2 -> Subsystem/2(Inport1)
  connections:
  Connection Port/RConn1 -- Three-Phase V-I Measurement/LConn1
  Connection Port1/RConn1 -- Three-Phase V-I Measurement/LConn2
  Connection Port2/RConn1 -- Three-Phase V-I Measurement/LConn3
  Connection Port4/RConn1 -- Three-Phase V-I Measurement/RConn1
  Three-Phase V-I Measurement/RConn2 -- Connection Port3/RConn1
  Three-Phase V-I Measurement/RConn3 -- Connection Port5/RConn1

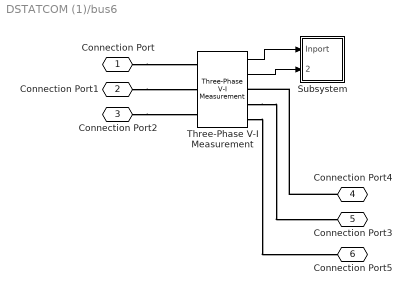
== system DSTATCOM (1)/bus6 ==
  Subsystem : Subsystem
  Three-Phase V-I Measurement : spsThreePhaseVIMeasurementLib/Three-Phase V-I Measurement  VoltageMeasurement=phase-to-ground  SetLabelV=off  LabelV=Vabc  Vpu=off  VpuLL=off  CurrentMeasurement=yes  SetLabelI=off  LabelI=Iabc  Ipu=off  Pbase=100e6  Vbase=500e3  OutputType=Complex  PhasorSimulation=off  PSBequivalent=0
  Connection Port : PMIOPort  Side=Left
  Connection Port1 : PMIOPort  Port=2  Side=Left
  Connection Port2 : PMIOPort  Port=3  Side=Left
  Connection Port4 : PMIOPort  Port=4  Side=Right
  Connection Port3 : PMIOPort  Port=5  Side=Right
  Connection Port5 : PMIOPort  Port=6  Side=Right
  wires:
  Three-Phase V-I Measurement/1 -> Subsystem/1(Inport)
  Three-Phase V-I Measurement/2 -> Subsystem/2(Inport1)
  connections:
  Connection Port/RConn1 -- Three-Phase V-I Measurement/LConn1
  Connection Port1/RConn1 -- Three-Phase V-I Measurement/LConn2
  Connection Port2/RConn1 -- Three-Phase V-I Measurement/LConn3
  Connection Port4/RConn1 -- Three-Phase V-I Measurement/RConn1
  Three-Phase V-I Measurement/RConn2 -- Connection Port3/RConn1
  Three-Phase V-I Measurement/RConn3 -- Connection Port5/RConn1

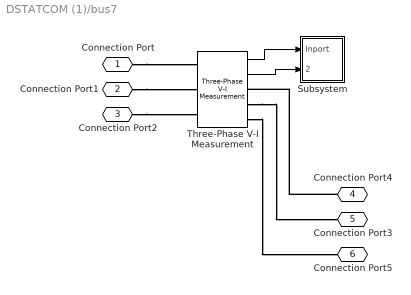
== system DSTATCOM (1)/bus7 ==
  Subsystem : Subsystem
  Three-Phase V-I Measurement : spsThreePhaseVIMeasurementLib/Three-Phase V-I Measurement  VoltageMeasurement=phase-to-ground  SetLabelV=off  LabelV=Vabc  Vpu=off  VpuLL=off  CurrentMeasurement=yes  SetLabelI=off  LabelI=Iabc  Ipu=off  Pbase=100e6  Vbase=500e3  OutputType=Complex  PhasorSimulation=off  PSBequivalent=0
  Connection Port : PMIOPort  Side=Left
  Connection Port1 : PMIOPort  Port=2  Side=Left
  Connection Port2 : PMIOPort  Port=3  Side=Left
  Connection Port4 : PMIOPort  Port=4  Side=Right
  Connection Port3 : PMIOPort  Port=5  Side=Right
  Connection Port5 : PMIOPort  Port=6  Side=Right
  wires:
  Three-Phase V-I Measurement/1 -> Subsystem/1(Inport)
  Three-Phase V-I Measurement/2 -> Subsystem/2(Inport1)
  connections:
  Connection Port/RConn1 -- Three-Phase V-I Measurement/LConn1
  Connection Port1/RConn1 -- Three-Phase V-I Measurement/LConn2
  Connection Port2/RConn1 -- Three-Phase V-I Measurement/LConn3
  Connection Port4/RConn1 -- Three-Phase V-I Measurement/RConn1
  Three-Phase V-I Measurement/RConn2 -- Connection Port3/RConn1
  Three-Phase V-I Measurement/RConn3 -- Connection Port5/RConn1

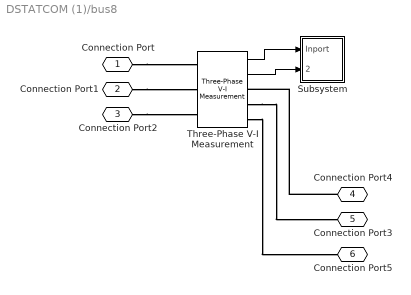
== system DSTATCOM (1)/bus8 ==
  Subsystem : Subsystem
  Three-Phase V-I Measurement : spsThreePhaseVIMeasurementLib/Three-Phase V-I Measurement  VoltageMeasurement=phase-to-ground  SetLabelV=off  LabelV=Vabc  Vpu=off  VpuLL=off  CurrentMeasurement=yes  SetLabelI=off  LabelI=Iabc  Ipu=off  Pbase=100e6  Vbase=500e3  OutputType=Complex  PhasorSimulation=off  PSBequivalent=0
  Connection Port : PMIOPort  Side=Left
  Connection Port1 : PMIOPort  Port=2  Side=Left
  Connection Port2 : PMIOPort  Port=3  Side=Left
  Connection Port4 : PMIOPort  Port=4  Side=Right
  Connection Port3 : PMIOPort  Port=5  Side=Right
  Connection Port5 : PMIOPort  Port=6  Side=Right
  wires:
  Three-Phase V-I Measurement/1 -> Subsystem/1(Inport)
  Three-Phase V-I Measurement/2 -> Subsystem/2(Inport1)
  connections:
  Connection Port/RConn1 -- Three-Phase V-I Measurement/LConn1
  Connection Port1/RConn1 -- Three-Phase V-I Measurement/LConn2
  Connection Port2/RConn1 -- Three-Phase V-I Measurement/LConn3
  Connection Port4/RConn1 -- Three-Phase V-I Measurement/RConn1
  Three-Phase V-I Measurement/RConn2 -- Connection Port3/RConn1
  Three-Phase V-I Measurement/RConn3 -- Connection Port5/RConn1

== system DSTATCOM (1)/bus9 ==
  Subsystem : Subsystem
  Three-Phase V-I Measurement : spsThreePhaseVIMeasurementLib/Three-Phase V-I Measurement  VoltageMeasurement=phase-to-ground  SetLabelV=off  LabelV=Vabc  Vpu=off  VpuLL=off  CurrentMeasurement=yes  SetLabelI=off  LabelI=Iabc  Ipu=off  Pbase=100e6  Vbase=500e3  OutputType=Complex  PhasorSimulation=off  PSBequivalent=0
  Connection Port : PMIOPort  Side=Left
  Connection Port1 : PMIOPort  Port=2  Side=Left
  Connection Port2 : PMIOPort  Port=3  Side=Left
  Connection Port4 : PMIOPort  Port=4  Side=Right
  Connection Port3 : PMIOPort  Port=5  Side=Right
  Connection Port5 : PMIOPort  Port=6  Side=Right
  wires:
  Three-Phase V-I Measurement/1 -> Subsystem/1(Inport)
  Three-Phase V-I Measurement/2 -> Subsystem/2(Inport1)
  connections:
  Connection Port/RConn1 -- Three-Phase V-I Measurement/LConn1
  Connection Port1/RConn1 -- Three-Phase V-I Measurement/LConn2
  Connection Port2/RConn1 -- Three-Phase V-I Measurement/LConn3
  Connection Port4/RConn1 -- Three-Phase V-I Measurement/RConn1
  Three-Phase V-I Measurement/RConn2 -- Connection Port3/RConn1
  Three-Phase V-I Measurement/RConn3 -- Connection Port5/RConn1

== system DSTATCOM (1)/load ==
  Subsystem : Subsystem
  Three-Phase V-I Measurement : spsThreePhaseVIMeasurementLib/Three-Phase V-I Measurement  VoltageMeasurement=phase-to-ground  SetLabelV=off  LabelV=Vabc  Vpu=off  VpuLL=off  CurrentMeasurement=yes  SetLabelI=off  LabelI=Iabc  Ipu=off  Pbase=100e6  Vbase=500e3  OutputType=Complex  PhasorSimulation=off  PSBequivalent=0
  Connection Port : PMIOPort  Side=Left
  Connection Port1 : PMIOPort  Port=2  Side=Left
  Connection Port2 : PMIOPort  Port=3  Side=Left
  Connection Port4 : PMIOPort  Port=4  Side=Right
  Connection Port3 : PMIOPort  Port=5  Side=Right
  Connection Port5 : PMIOPort  Port=6  Side=Right
  wires:
  Three-Phase V-I Measurement/1 -> Subsystem/1(Inport)
  Three-Phase V-I Measurement/2 -> Subsystem/2(Inport1)
  connections:
  Connection Port/RConn1 -- Three-Phase V-I Measurement/LConn1
  Connection Port1/RConn1 -- Three-Phase V-I Measurement/LConn2
  Connection Port2/RConn1 -- Three-Phase V-I Measurement/LConn3
  Connection Port4/RConn1 -- Three-Phase V-I Measurement/RConn1
  Three-Phase V-I Measurement/RConn2 -- Connection Port3/RConn1
  Three-Phase V-I Measurement/RConn3 -- Connection Port5/RConn1

== system DSTATCOM (1)/source ==
  Three-Phase V-I Measurement : spsThreePhaseVIMeasurementLib/Three-Phase V-I Measurement  VoltageMeasurement=phase-to-ground  SetLabelV=off  LabelV=Vabc  Vpu=off  VpuLL=off  CurrentMeasurement=yes  SetLabelI=off  LabelI=Iabc  Ipu=off  Pbase=100e6  Vbase=500e3  OutputType=Complex  PhasorSimulation=off  PSBequivalent=0
  vi : Subsystem
  inphase a : PMIOPort  Side=Left
  inphase b : PMIOPort  Port=2  Side=Left
  inphase c : PMIOPort  Port=3  Side=Left
  outphase a : PMIOPort  Port=4  Side=Right
  outphase b : PMIOPort  Port=5  Side=Right
  outphase c : PMIOPort  Port=6  Side=Right
  wires:
  Three-Phase V-I Measurement/1 -> vi/1(Inport)
  Three-Phase V-I Measurement/2 -> vi/2(Inport1)
  connections:
  inphase a/RConn1 -- Three-Phase V-I Measurement/LConn1
  inphase b/RConn1 -- Three-Phase V-I Measurement/LConn2
  inphase c/RConn1 -- Three-Phase V-I Measurement/LConn3
  outphase a/RConn1 -- Three-Phase V-I Measurement/RConn1
  Three-Phase V-I Measurement/RConn2 -- outphase b/RConn1
  Three-Phase V-I Measurement/RConn3 -- outphase c/RConn1

== system DSTATCOM (1)/Iinv/Subsystem ==
  Inport : Inport
  Inport1 : Inport  Port=2
  tag scope: Iinv=global, Vinv=global
  wires:
  Inport/1 -> [Vinv]
  Inport1/1 -> [Iinv]

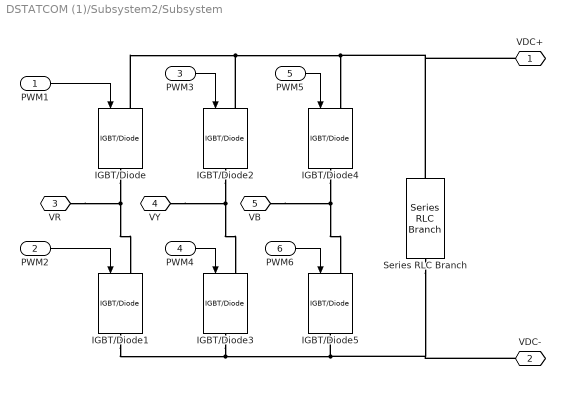
== system DSTATCOM (1)/Subsystem2/Subsystem ==
  PWM1 : Inport
  PWM2 : Inport  Port=2
  PWM3 : Inport  Port=3
  PWM4 : Inport  Port=4
  PWM5 : Inport  Port=5
  PWM6 : Inport  Port=6
  IGBT/Diode{,1..5} (6 alike) : spsIGBTDiodeLib/IGBT//Diode  Ron=1e-3  Rs=1e5  Cs=inf  Measurements=off
  Series RLC Branch : spsSeriesRLCBranchLib/Series RLC Branch  LConnTagsString=__new0  RConnTagsString=__new0  BranchType=RC  Resistance=1e-3  Inductance=1e-3  SetiL0=off  InitialCurrent=0  Capacitance=5600e-6  Setx0=off  InitialVoltage=0  Measurements=None
  VDC+ : PMIOPort  Side=Right
  VDC- : PMIOPort  Port=2  Side=Right
  VR : PMIOPort  Port=3  Side=Left
  VY : PMIOPort  Port=4  Side=Left
  VB : PMIOPort  Port=5  Side=Left
  wires:
  PWM2/1 -> IGBT/Diode1/1
  PWM6/1 -> IGBT/Diode5/1
  PWM1/1 -> IGBT/Diode/1
  PWM5/1 -> IGBT/Diode4/1
  PWM3/1 -> IGBT/Diode2/1
  PWM4/1 -> IGBT/Diode3/1
  connections:
  IGBT/Diode1/RConn1 -- IGBT/Diode3/RConn1 -- VDC-/RConn1 -- Series RLC Branch/RConn1 -- IGBT/Diode5/RConn1
  IGBT/Diode/LConn1 -- IGBT/Diode2/LConn1 -- VDC+/RConn1 -- Series RLC Branch/LConn1 -- IGBT/Diode4/LConn1
  IGBT/Diode4/RConn1 -- VB/RConn1 -- IGBT/Diode5/LConn1
  IGBT/Diode2/RConn1 -- VY/RConn1 -- IGBT/Diode3/LConn1
  IGBT/Diode/RConn1 -- VR/RConn1 -- IGBT/Diode1/LConn1

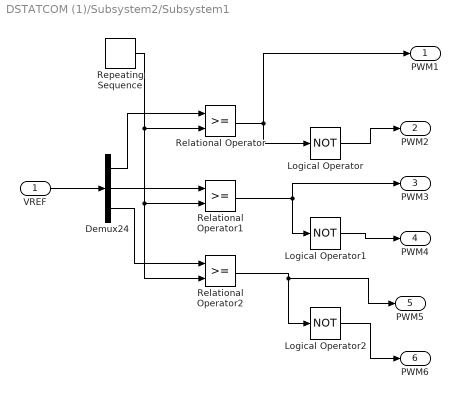
== system DSTATCOM (1)/Subsystem2/Subsystem1 ==
  VREF : Inport
  Demux24 : Demux  Outputs=3
  Logical Operator : Logic  Operator=NOT  AllPortsSameDT=off  OutDataTypeStr=boolean
  Logical Operator1 : Logic  Operator=NOT  AllPortsSameDT=off  OutDataTypeStr=boolean
  Logical Operator2 : Logic  Operator=NOT  AllPortsSameDT=off  OutDataTypeStr=boolean
  Relational Operator : RelationalOperator  OutDataTypeStr=boolean  RndMeth=Simplest  InputSameDT=off
  Relational Operator1 : RelationalOperator  OutDataTypeStr=boolean  RndMeth=Simplest  InputSameDT=off
  Relational Operator2 : RelationalOperator  OutDataTypeStr=boolean  RndMeth=Simplest  InputSameDT=off
  Repeating Sequence : simulink/Sources/Repeating Sequence  rep_seq_t=[0 0.0005 0.001]  rep_seq_y=[-1 0 -1]
  PWM1 : Outport
  PWM2 : Outport  Port=2
  PWM3 : Outport  Port=3
  PWM4 : Outport  Port=4
  PWM5 : Outport  Port=5
  PWM6 : Outport  Port=6
  wires:
  Relational Operator1/1 -> PWM3/1, Logical Operator1/1
  VREF/1 -> Demux24/1
  Relational Operator/1 -> PWM1/1, Logical Operator/1
  Logical Operator/1 -> PWM2/1
  Demux24/3 -> Relational Operator2/1
  Logical Operator1/1 -> PWM4/1
  Relational Operator2/1 -> PWM5/1, Logical Operator2/1
  Demux24/1 -> Relational Operator/1
  Repeating Sequence/1 -> Relational Operator2/2, Relational Operator1/2, Relational Operator/2
  Logical Operator2/1 -> PWM6/1
  Demux24/2 -> Relational Operator1/1

== system DSTATCOM (1)/bus10/Subsystem ==
  Inport : Inport
  Inport1 : Inport  Port=2
  tag scope: I10ABC=global, V10ABC=global
  wires:
  Inport/1 -> [V10ABC]
  Inport1/1 -> [I10ABC]

== system DSTATCOM (1)/bus2/Subsystem ==
  Inport : Inport
  Inport1 : Inport  Port=2
  tag scope: I2ABC=global, V2ABC=global
  wires:
  Inport/1 -> [V2ABC]
  Inport1/1 -> [I2ABC]

== system DSTATCOM (1)/bus3/Subsystem ==
  Inport : Inport
  Inport1 : Inport  Port=2
  tag scope: I3ABC=global, V3ABC=global
  wires:
  Inport/1 -> [V3ABC]
  Inport1/1 -> [I3ABC]

== system DSTATCOM (1)/bus5/Subsystem ==
  Inport : Inport
  Inport1 : Inport  Port=2
  tag scope: I5ABC=global, V5ABC=global
  wires:
  Inport/1 -> [V5ABC]
  Inport1/1 -> [I5ABC]

== system DSTATCOM (1)/bus6/Subsystem ==
  Inport : Inport
  Inport1 : Inport  Port=2
  tag scope: I6ABC=global, V6ABC=global
  wires:
  Inport/1 -> [V6ABC]
  Inport1/1 -> [I6ABC]

== system DSTATCOM (1)/bus7/Subsystem ==
  Inport : Inport
  Inport1 : Inport  Port=2
  tag scope: I7ABC=global, V7ABC=global
  wires:
  Inport/1 -> [V7ABC]
  Inport1/1 -> [I7ABC]

== system DSTATCOM (1)/bus8/Subsystem ==
  Inport : Inport
  Inport1 : Inport  Port=2
  tag scope: I8ABC=global, V8ABC=global
  wires:
  Inport/1 -> [V8ABC]
  Inport1/1 -> [I8ABC]

== system DSTATCOM (1)/bus9/Subsystem ==
  Inport : Inport
  Inport1 : Inport  Port=2
  tag scope: I9ABC=global, V9ABC=global
  wires:
  Inport/1 -> [V9ABC]
  Inport1/1 -> [I9ABC]

== system DSTATCOM (1)/load/Subsystem ==
  Inport : Inport
  Inport1 : Inport  Port=2
  tag scope: Iload=global, Vload=global
  wires:
  Inport/1 -> [Vload]
  Inport1/1 -> [Iload]

== system DSTATCOM (1)/source/vi ==
  Inport : Inport
  Inport1 : Inport  Port=2
  tag scope: Iabc=global, Vabc=global
  wires:
  Inport/1 -> [Vabc]
  Inport1/1 -> [Iabc]
